simulink model "ue1simulink"  (R2020b)
settings: Solver=VariableStepAuto  StartTime=0.0  StopTime=25  RelTol=1e-3
values from neighbouring files (symbols this model uses):
  C = 100*1e-6    (= 0.0001)    [test_ue1.m]
  R = real(P)    [myisstable.m]    (also in polvorgabe.m = P; polvorgabe_HStoerung.m = tf(b, a); polvorgabe_zusatz.m = tf(b, a); resultante.m = a(1:end, 1:dim2))
  Uin = 2    [test_ue1.m]
libraries: cstblocks x1
settings Model: Creator=valnim  LastModifiedBy=valnim

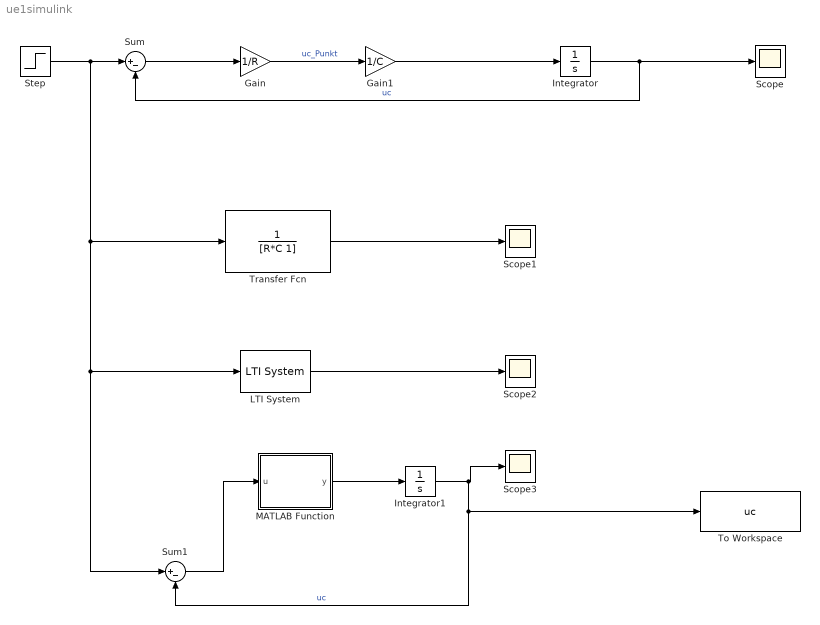
== system ue1simulink ==
  Gain : Gain  Gain=1/R
  Gain1 : Gain  Gain=1/C
  Integrator : Integrator
  Integrator1 : Integrator
  LTI System : cstblocks/LTI System  sys=P  IC=[]
  MATLAB Function : MATLAB Function  TreatAsAtomicUnit=on
  Scope{,1..3} (4 alike) : Scope
  Step : Step  After=Uin  SampleTime=0
  Sum : Sum  Inputs=|+-
  Sum1 : Sum  Inputs=|+-
  To Workspace : ToWorkspace  VariableName=uc  SaveFormat=Timeseries  SampleTime=-1
  Transfer Fcn : TransferFcn  Denominator=[R*C 1]
  wires:
  Gain1/1 -> Integrator/1
  Gain/1 -> Gain1/1  "uc_Punkt"
  Integrator/1 -> Sum/2, Scope/1  "uc"
  Sum/1 -> Gain/1
  Transfer Fcn/1 -> Scope1/1
  Step/1 -> Sum1/1, LTI System/1, Transfer Fcn/1, Sum/1
  LTI System/1 -> Scope2/1
  MATLAB Function/1(y) -> Integrator1/1
  Integrator1/1 -> Sum1/2, To Workspace/1, Scope3/1  "uc"
  Sum1/1 -> MATLAB Function/1(u)

== matlab function ue1simulink/MATLAB Function ==
  data: y output; u input; R parameter; C parameter
function y = fcn(u, R, C)
    
y = 1/(R*C)*u;
